simulink model "Project"  (R2024a)
settings: Solver=VariableStepAuto  StartTime=0.0  StopTime=10.0  RelTol=1e-3
values from neighbouring files (symbols this model uses):
  B = 0.02    [Script.m]
  J = 7    [Script.m]
  K = 1.4    [Script.m]
  La = 0.4    [Script.m]
  Ra = 0.4    [Script.m]
  Tl = 30    [Script.m]
  Va = 100    [Script.m]

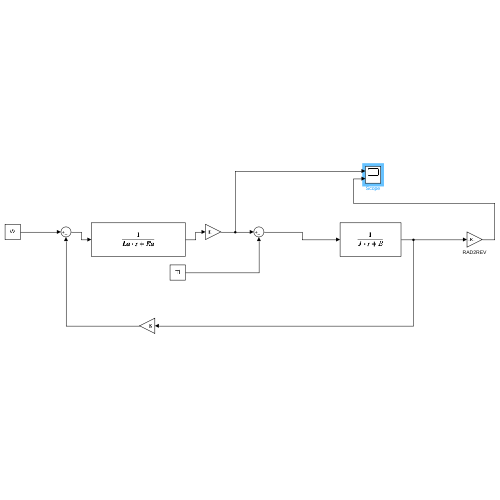
[thumbnail: Simulink's stored preview of the top-level diagram]
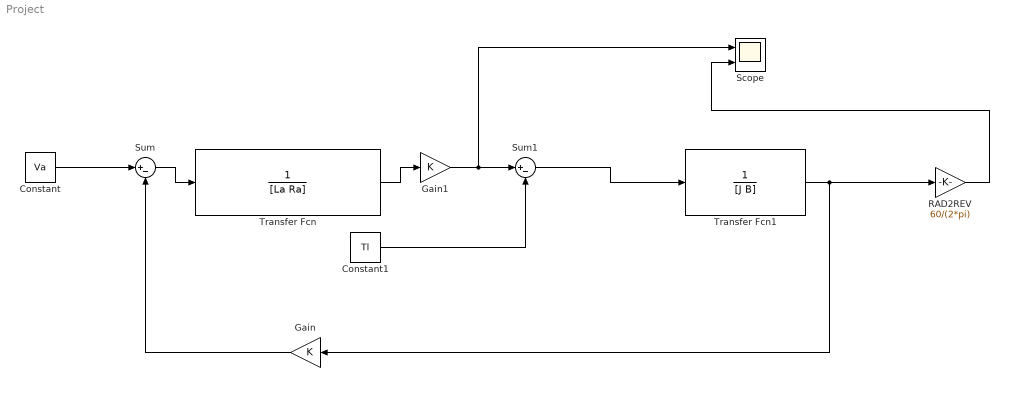
== system Project ==
  Constant : Constant  Value=Va
  Constant1 : Constant  Value=Tl
  Gain : Gain  Gain=K
  Gain1 : Gain  Gain=K
  RAD2REV : Gain  Gain=60/(2*pi)
  Scope : Scope  NumInputPorts=2
  Sum : Sum  Inputs=|+-
  Sum1 : Sum  Inputs=|+-
  Transfer Fcn : TransferFcn  Denominator=[La Ra]
  Transfer Fcn1 : TransferFcn  Denominator=[J B]
  wires:
  Constant/1 -> Sum/1
  Sum/1 -> Transfer Fcn/1
  Gain/1 -> Sum/2
  Transfer Fcn/1 -> Gain1/1
  Gain1/1 -> Scope/1, Sum1/1
  Sum1/1 -> Transfer Fcn1/1
  Constant1/1 -> Sum1/2
  Transfer Fcn1/1 -> RAD2REV/1, Gain/1
  RAD2REV/1 -> Scope/2
